simulink model "PR_controlv8planning"  (R2024a)
settings: Solver=VariableStepAuto  StartTime=0.0  StopTime=stoptime  RelTol=1e-3
values from neighbouring files (symbols this model uses):
  amp_factor = 0.01    [find_different_length_masses.m]    (also in find_different_length_masses_noretrain.m; find_good_reservoirs.m; plot_angle.m)
  rc = ESN_trainbysim(Nr, 'sizeinput', sizeinput, 'nodenuminput', 3, 'sizeoutput', sizeoutput,              'timeConst', timeConstant, 'spectralRadius', SR, 'inputScaling', 1, 'connectivity', 0.5, 'biasScaling', 0,              'regularization', 1e-1, 'delaylen', 0.1, 'timestep', 0.01, 'normmethod', normmethod, 'ifxnorm', ifxnorm, 'sizereadout', Nr + sizeinput + 1)    [find_different_length_masses.m]    (also in find_different_length_masses_noretrain.m; find_good_reservoirs.m = ESN_trainbysim(Nr, 'sizeinput', sizeinput, 'nodenuminput', 3; plot_angle.m)
  robot_pendepth = 0.02    [find_different_length_masses.m]    (also in find_different_length_masses_noretrain.m; find_good_reservoirs.m; plot_angle.m)
  robot_penlength = 0.2    [find_different_length_masses.m]    (also in find_different_length_masses_noretrain.m; find_good_reservoirs.m; plot_angle.m = 0.1)
  robot_penwidth = 0.02    [find_different_length_masses.m]    (also in find_different_length_masses_noretrain.m; find_good_reservoirs.m; plot_angle.m)
  robot_sphere_mass = 0.1    [find_different_length_masses.m]    (also in find_different_length_masses_noretrain.m; find_good_reservoirs.m; plot_angle.m)
  samplingrate = 0.01    [find_different_length_masses.m]    (also in find_different_length_masses_noretrain.m; find_good_reservoirs.m; plot_angle.m; stmpcevaluation.m)
  torquelim = fraction*mass*robot_penlength    (= 0.05)    [find_different_length_masses.m]    (also in find_different_length_masses_noretrain.m; find_good_reservoirs.m; plot_angle.m)
  Win = eye(2)    [find_different_length_masses.m]    (also in find_different_length_masses_noretrain.m; find_good_reservoirs.m; plot_angle.m; stmpcevaluation.m)
  X = esn.train_reservoirReadoutWashed    [ESN_trainbysim.m]
  Y = esn.train_reservoirTargetWashed{i}    [ESN_trainbysim.m]
undefined symbols (not defined in the file or in its folder): arm_radius, arm_radius_previus, spring_position_scale, Z
libraries: sm_lib x9, nesl_utility x5, dspindex x1
settings Model: Creator=fy264  LastModifiedBy=fy264
settings OptimizationCC: ReuseModelBlockBuffer=off
settings DebuggingCC: AlgebraicLoopMsg=none  ArtificialAlgebraicLoopMsg=none
settings RTWCC: GPUComputeCapability=3.5

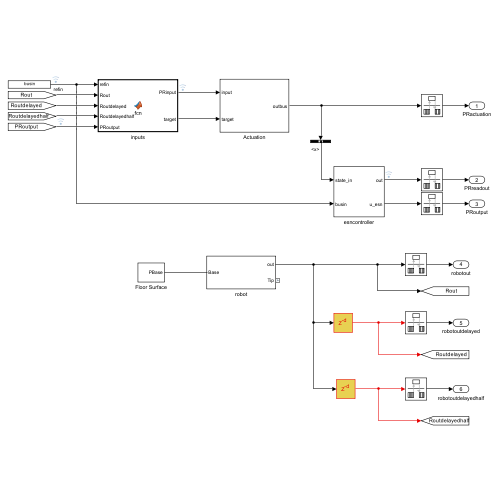
[thumbnail: Simulink's stored preview of the top-level diagram]
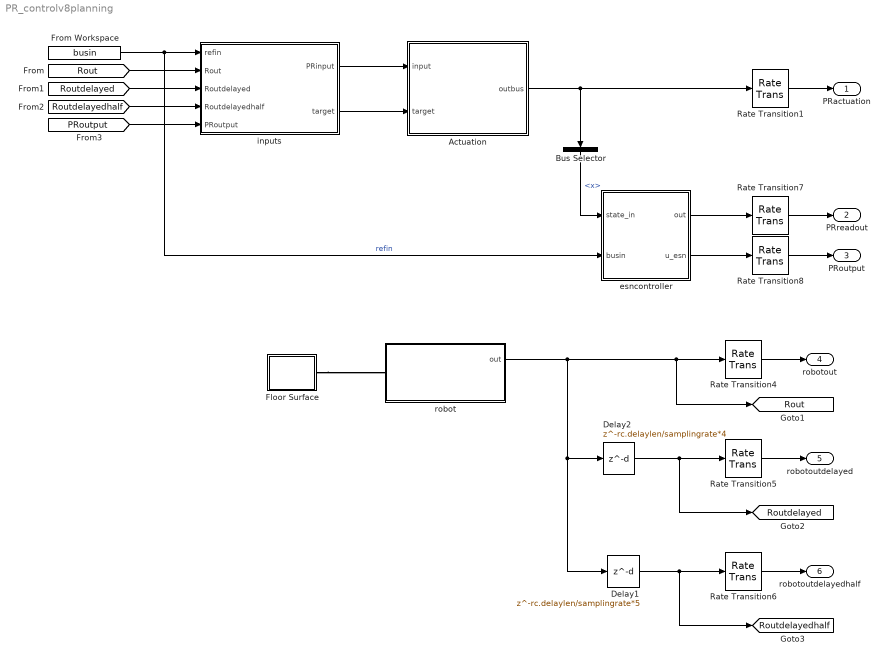
== system PR_controlv8planning ==
  Actuation : Subsystem  mask{xnorm=rc.xnorm}
  Bus Selector : BusSelector  OutputSignals=x
  Delay1 : Delay  DelayLength=rc.delaylen/samplingrate*5  InitialCondition=0
  Delay2 : Delay  DelayLength=rc.delaylen/samplingrate*4  InitialCondition=0
  Floor Surface : Subsystem  mask{length=0.5, width=0.5}
      mask prompts: length "grid length [m]"; width "grid width [m]"
  From Workspace : FromWorkspace  VariableName=busin  OutDataTypeStr=Bus: SinusoidBus  OutputAfterFinalValue=Holding final value
  Rate Transition{1,4..8} (6 alike) : RateTransition  OutPortSampleTime=samplingrate
  esncontroller : Subsystem  mask{Nr=rc.Nr, tau=rc.tau, Win=rc.Win, Wb=rc.Wb, Wr=rc.Wr, sizeinput=rc.sizeinput, nodenuminput=rc.nodenuminput, timestep=rc.timestep, ini_S=rc.initialstate, delaylen=rc.delaylen, delaynorm=rc.delaynorm, normmethod=rc.normmethod, ifxnorm=rc.ifxnorm, xnorm=rc.xnorm, Wout=0}
      mask prompts: delaynorm "delaynrom"
  inputs : MATLAB Function  TreatAsAtomicUnit=on
  robot : Subsystem
  PRactuation : Outport
  PRreadout : Outport  Port=2
  PRoutput : Outport  Port=3
  robotout : Outport  Port=4
  robotoutdelayed : Outport  Port=5
  robotoutdelayedhalf : Outport  Port=6
  tag scope: Rout=global, Routdelayed=global, Routdelayedhalf=global
  wires:
  Actuation/1(outbus) -> Bus Selector/1, Rate Transition1/1
  Rate Transition1/1 -> PRactuation/1
  Rate Transition4/1 -> robotout/1
  inputs/1(PRinput) -> Actuation/1(input)
  From Workspace/1 -> esncontroller/2(busin), inputs/1(refin)  "refin"
  [Rout] -> inputs/2(Rout)
  Rate Transition5/1 -> robotoutdelayed/1
  robot/1(out) -> Delay2/1, Delay1/1, Rate Transition4/1, [Rout]
  Delay2/1 -> [Routdelayed], Rate Transition5/1
  [Routdelayed] -> inputs/3(Routdelayed)
  inputs/2(target) -> Actuation/2(target)
  Delay1/1 -> [Routdelayedhalf], Rate Transition6/1
  Rate Transition6/1 -> robotoutdelayedhalf/1
  [Routdelayedhalf] -> inputs/4(Routdelayedhalf)
  esncontroller/2(u_esn) -> Rate Transition8/1
  Bus Selector/1 -> esncontroller/1(state_in)  "<x>"
  esncontroller/1(out) -> Rate Transition7/1
  Rate Transition7/1 -> PRreadout/1
  Rate Transition8/1 -> PRoutput/1
  [PRoutput] -> inputs/5(PRoutput)
  connections:
  Floor Surface/RConn1 -- robot/LConn1

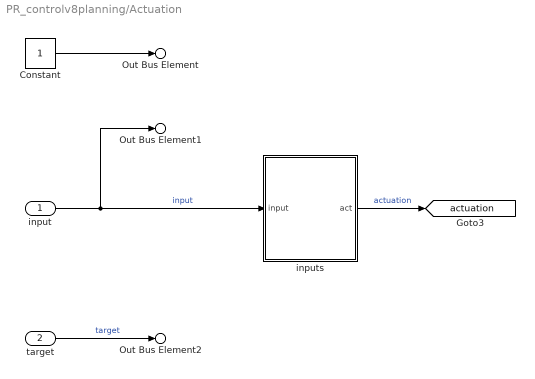
== system PR_controlv8planning/Actuation ==
  input : Inport
  target : Inport  Port=2
  Constant : Constant
  inputs : MATLAB Function  TreatAsAtomicUnit=on
  Out Bus Element : Outport  PortName=outbus  Element=const
  Out Bus Element1 : Outport  PortName=outbus  Element=x
  Out Bus Element2 : Outport  PortName=outbus  Element=target
  tag scope: actuation=global
  wires:
  input/1 -> Out Bus Element1/1, inputs/1(input)  "input"
  inputs/1(act) -> [actuation]  "actuation"
  Constant/1 -> Out Bus Element/1
  target/1 -> Out Bus Element2/1  "target"

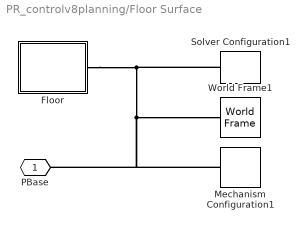
== system PR_controlv8planning/Floor Surface ==
  Floor : Subsystem
  Mechanism Configuration1 : sm_lib/Utilities/Mechanism Configuration  UniformGravity=Constant  GravityVector=[0 0 -9.80665]  GravityVectorUnits=m/s^2  LinearizationDelta=0.001  JointModeTransitionNonlinearIterations=2
  Solver Configuration1 : nesl_utility/Solver Configuration  PhysicalDomain=network_engine_domain  SubClassName=solver  LeftPortType=input  RightPortType=generic  Tones=[]  Harmonics=[]  SimulateNoise=off  Profile=off  UseLocalSampling=off  EnableSwitchedLinearOptims=on  FrequencyDomain=off  UseCCode=off  RelTol=0.001  AbsTol=1e-06  MinStep=1e-09  ToWorkspace=off  RevertToSquareIcSolve=off  NumHomotopyIterations=100  PhasorMode=off  PhasorModeNumHarmonics=1  ConsistencySolver=NEWTON_FTOL  IndexReductionMethod=DerivativeReplacement  DoDC=off  ResidualTolerance=1e-09  ConsistencyTolSource=GLOBAL  ConsistencyAbsTol=0.001  ConsistencyRelTol=0.001  ConsistencyTolFactor=0.001  UseLocalSolver=off  LocalSolverChoice=NE_BACKWARD_EULER_ADVANCER  ResolveIndetEquations=on  FunctionEvalNumThread=1  LocalSolverSampleTime=0.0002  DoFixedCost=off  MaxNonlinIter=10  MaxModeIter=2  ComputeImpulses=off  ImpulseIterations=2  LinearAlgebra=Sparse  LinearAlgebraNumThread=0  EquationFormulation=NE_TIME_EF  DelaysMemoryBudget=1024  AutomaticFiltering=off  FilteringTimeConstant=0.001  PartitionStorageMethod=AS_NEEDED  PartitionMemoryBudget=1024  PartitionMethod=FAST  MultibodyUseLocalSolver=off  MultibodyLocalSolverChoice=ODE1  MultibodyLocalSolverSampleTime=0.001
  World Frame1 : sm_lib/Frames and Transforms/World Frame
  PBase : PMIOPort  Side=Right
  connections:
  Floor/RConn1 -- PBase/RConn1 -- Mechanism Configuration1/RConn1 -- World Frame1/RConn1 -- Solver Configuration1/RConn1

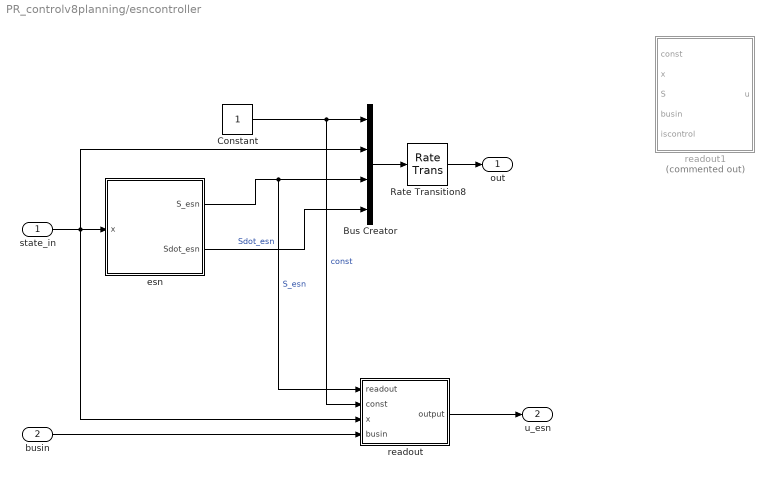
== system PR_controlv8planning/esncontroller ==
  state_in : Inport
  busin : Inport  Port=2
  Bus Creator : BusCreator  Inputs=4
  Constant : Constant
  Rate Transition8 : RateTransition  OutPortSampleTime=timestep
  esn : Subsystem  mask{Nr=rc.Nr, sizeinput=rc.sizeinput, nodenuminput=rc.nodenuminput, Win=rc.Win, Wr=rc.Wr, Wb=rc.Wb, tau=rc.tau, timestep=rc.timestep, ini_S=rc.initialstate}
  readout : Subsystem  mask{Woutmat=rc.Woutmat}
  readout1 : MATLAB Function  Commented=on  TreatAsAtomicUnit=on
  out : Outport
  u_esn : Outport  Port=2
  wires:
  Bus Creator/1 -> Rate Transition8/1
  Rate Transition8/1 -> out/1
  esn/2(Sdot_esn) -> Bus Creator/4  "Sdot_esn"
  esn/1(S_esn) -> readout/1(readout), Bus Creator/3  "S_esn"
  Constant/1 -> readout/2(const), Bus Creator/1  "const"
  state_in/1 -> readout/3(x), esn/1(x), Bus Creator/2
  busin/1 -> readout/4(busin)
  readout/1(output) -> u_esn/1

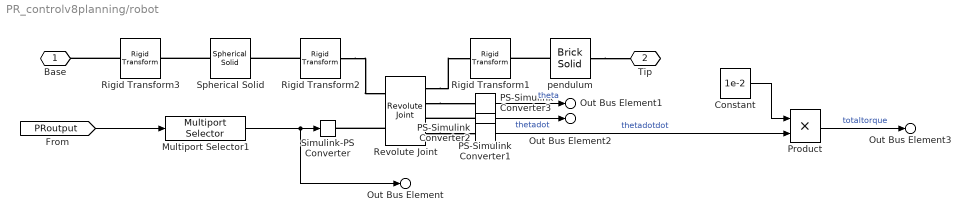
== system PR_controlv8planning/robot ==
  Constant : Constant  Value=1e-2
  Multiport Selector1 : dspindex/Multiport Selector  rowsOrCols=Rows  idxCellArray=1  idxErrMode=Clip Index
  PS-Simulink Converter1 : nesl_utility/PS-Simulink Converter  PhysicalDomain=network_engine_domain  SubClassName=ps_output  LeftPortType=input  RightPortType=output  PseudoPeriodic=off  Frequencies=[]  VectorFormat=1-D array  Unit=1  AffineConversion=off
  PS-Simulink Converter2 : nesl_utility/PS-Simulink Converter  PhysicalDomain=network_engine_domain  SubClassName=ps_output  LeftPortType=input  RightPortType=output  PseudoPeriodic=off  Frequencies=[]  VectorFormat=1-D array  Unit=1  AffineConversion=off
  PS-Simulink Converter3 : nesl_utility/PS-Simulink Converter  PhysicalDomain=network_engine_domain  SubClassName=ps_output  LeftPortType=input  RightPortType=output  PseudoPeriodic=off  Frequencies=[]  VectorFormat=1-D array  Unit=1  AffineConversion=off
  Product : Product
  Revolute Joint : sm_lib/Joints/Revolute Joint  JointMode=Normal  CompositeWrenchDir=FollowerOnBase  CompositeWrenchFrame=BaseFrame  SenseConstraintForce=off  SenseConstraintTorque=off  SenseTotalForce=off  SenseTotalTorque=off  PositionTargetSpecify=on  PositionTargetPriority=Low  PositionTargetValue=robot_ini_theta_p  PositionTargetValueUnits=rad  VelocityTargetSpecify=on  VelocityTargetPriority=Low  VelocityTargetValue=robot_ini_thetadot_p  VelocityTargetValueUnits=rad/s  EquilibriumPosition=0  EquilibriumPositionUnits=rad  SpringStiffness=0  SpringStiffnessUnits=N*m/rad  DampingCoefficient=robot_damping_coeff  DampingCoefficientUnits=N*m/(rad/s)  LowerLimitSpecify=off  LowerLimitBound=-90  LowerLimitBoundUnits=deg  LowerLimitStiffness=1e4  LowerLimitStiffnessUnits=N*m/deg  LowerLimitDamping=10  LowerLimitDampingUnits=N*m/(deg/s)  LowerLimitTransitionRegionWidth=0.1  LowerLimitTransitionRegionWidthUnits=deg  UpperLimitSpecify=off  UpperLimitBound=90  UpperLimitBoundUnits=deg  UpperLimitStiffness=1e4  UpperLimitStiffnessUnits=N*m/deg  UpperLimitDamping=10  UpperLimitDampingUnits=N*m/(deg/s)  UpperLimitTransitionRegionWidth=0.1  UpperLimitTransitionRegionWidthUnits=deg  TorqueActuationMode=InputTorque  MotionActuationMode=ComputedMotion  SensePosition=on  SenseVelocity=on  SenseAcceleration=on  SenseTorqueForce=off  SenseLowerLimitTorqueForce=off  SenseUpperLimitTorqueForce=off
  Rigid Transform1 : sm_lib/Frames and Transforms/Rigid Transform  RotationMethod=AlignedAxes  FollAlignAxisA=+X  BaseAlignAxisA=+X  FollAlignAxisB=-Z  BaseAlignAxisB=+Y  RotationStandardAxis=+Z  RotationAngle=180  RotationAngleUnits=deg  RotationArbitraryAxis=[0 0 1]  RotationSequenceAxes=FollowerAxes  RotationSequence=XYX  RotationSequenceAngles=[0 0 0]  RotationSequenceAnglesUnits=deg  RotationMatrix=[1 0 0; 0 1 0; 0 0 1]  Quaternion=[1 0 0 0]  TranslationMethod=None  TranslationCartesianOffset=[arm_radius*spring_position_scale 0 0]  TranslationCartesianOffsetUnits=m  TranslationStandardAxis=+Z  TranslationStandardOffset=0  TranslationStandardOffsetUnits=m  TranslationROffset=arm_radius_previus*spring_position_scale  TranslationROffsetUnits=m  TranslationThetaOffset=theta  TranslationThetaOffsetUnits=deg  TranslationZOffset=0  TranslationZOffsetUnits=m
  Rigid Transform2 : sm_lib/Frames and Transforms/Rigid Transform  RotationMethod=AlignedAxes  FollAlignAxisA=+X  BaseAlignAxisA=+X  FollAlignAxisB=+Y  BaseAlignAxisB=+Z  RotationStandardAxis=+Z  RotationAngle=180  RotationAngleUnits=deg  RotationArbitraryAxis=[0 0 1]  RotationSequenceAxes=FollowerAxes  RotationSequence=XYX  RotationSequenceAngles=[0 0 0]  RotationSequenceAnglesUnits=deg  RotationMatrix=[1 0 0; 0 1 0; 0 0 1]  Quaternion=[1 0 0 0]  TranslationMethod=None  TranslationCartesianOffset=[arm_radius*spring_position_scale 0 0]  TranslationCartesianOffsetUnits=m  TranslationStandardAxis=+Z  TranslationStandardOffset=0  TranslationStandardOffsetUnits=m  TranslationROffset=arm_radius_previus*spring_position_scale  TranslationROffsetUnits=m  TranslationThetaOffset=theta  TranslationThetaOffsetUnits=deg  TranslationZOffset=0  TranslationZOffsetUnits=m
  Rigid Transform3 : sm_lib/Frames and Transforms/Rigid Transform  RotationMethod=None  FollAlignAxisA=+X  BaseAlignAxisA=+X  FollAlignAxisB=+Y  BaseAlignAxisB=+Z  RotationStandardAxis=+Z  RotationAngle=180  RotationAngleUnits=deg  RotationArbitraryAxis=[0 0 1]  RotationSequenceAxes=FollowerAxes  RotationSequence=XYX  RotationSequenceAngles=[0 0 0]  RotationSequenceAnglesUnits=deg  RotationMatrix=[1 0 0; 0 1 0; 0 0 1]  Quaternion=[1 0 0 0]  TranslationMethod=StandardAxis  TranslationCartesianOffset=[arm_radius*spring_position_scale 0 0]  TranslationCartesianOffsetUnits=m  TranslationStandardAxis=+Z  TranslationStandardOffset=robot_penposz  TranslationStandardOffsetUnits=m  TranslationROffset=arm_radius_previus*spring_position_scale  TranslationROffsetUnits=m  TranslationThetaOffset=theta  TranslationThetaOffsetUnits=deg  TranslationZOffset=0  TranslationZOffsetUnits=m
  Simulink-PS Converter : nesl_utility/Simulink-PS Converter  PhysicalDomain=network_engine_domain  SubClassName=ps_input  LeftPortType=input  RightPortType=output  PseudoPeriodic=off  Frequencies=[]  NoiseDistribution=none  NoiseParameters=[]  Unit=1  AffineConversion=off  FilteringAndDerivatives=provide  SimscapeFilterOrder=1  InputFilterTimeConstant=0.001  UdotUserProvided=0
  Spherical Solid : sm_lib/Body Elements/Spherical Solid  SphereRadius=robot_sphere_radius  SphereRadiusUnits=m  ExportEntireGeometry=off  InertiaType=CalculateFromGeometry  BasedOnType=Mass  Density=1000  DensityUnits=kg/m^3  Mass=robot_sphere_mass  MassUnits=kg  CenterOfMass=[0 0 0]  CenterOfMassUnits=m  MomentsOfInertia=[1 1 1]  MomentsOfInertiaUnits=kg*m^2  ProductsOfInertia=[0 0 0]  ProductsOfInertiaUnits=kg*m^2  GraphicType=FromGeometry  MarkerShape=Sphere  MarkerSize=10  GraphicVisPropType=SimpleVisualProperties  GraphicDiffuseColor=[1.0 0.0 0.0]  GraphicOpacity=1.0  GraphicSpecularColor=[0.5 0.5 0.5 1.0]  GraphicAmbientColor=[0.15 0.15 0.15 1.0]  GraphicEmissiveColor=[0.0 0.0 0.0 1.0]  GraphicShininess=75  DoExposeReferenceFrame=on  SerializedFrames=<Frames><Frame><Id>Frame1</Id><Value><Name>F1</Name><Origin><Source>ReferenceFrame</Source><FeatureName></FeatureName></Origin><PrimaryAxis><DefinedDirection>+Z</DefinedDirection><Source>ReferenceFrame</Source><SourceDirection>+Z</SourceDirection><FeatureName></FeatureName></PrimaryAxis><SecondaryAxis><DefinedDirection>+X</DefinedDirection><Source>ReferenceFrame</Source><SourceDirection>+X</SourceDirection><FeatureName></FeatureName></SecondaryAxis></Value></Frame></Frames>
  pendulum : sm_lib/Body Elements/Brick Solid  BrickDimensions=[robot_penwidth robot_pendepth robot_penlength]  BrickDimensionsUnits=m  ExportEntireGeometry=off  InertiaType=CalculateFromGeometry  BasedOnType=Density  Density=robot_penrho  DensityUnits=kg/m^3  Mass=1  MassUnits=kg  CenterOfMass=[0 0 0]  CenterOfMassUnits=m  MomentsOfInertia=[1 1 1]  MomentsOfInertiaUnits=kg*m^2  ProductsOfInertia=[0 0 0]  ProductsOfInertiaUnits=kg*m^2  GraphicType=FromGeometry  MarkerShape=Sphere  MarkerSize=10  GraphicVisPropType=SimpleVisualProperties  GraphicDiffuseColor=[1.0 0.0 1.0]  GraphicOpacity=1.0  GraphicSpecularColor=[0.5 0.5 0.5 1.0]  GraphicAmbientColor=[0.15 0.15 0.15 1.0]  GraphicEmissiveColor=[0.0 0.0 0.0 1.0]  GraphicShininess=75  DoExposeReferenceFrame=off  SerializedFrames=<Frames><Frame><Id>Frame1</Id><Value><Name>F1</Name><Origin><Source>GeometricFeature</Source><FeatureName>-z surface</FeatureName></Origin><PrimaryAxis><DefinedDirection>+Z</DefinedDirection><Source>ReferenceFrame</Source><SourceDirection>+Z</SourceDirection><FeatureName></FeatureName></PrimaryAxis><SecondaryAxis><DefinedDirection>+X</DefinedDirection><Source>ReferenceFrame</Source><SourceDirection>+X</SourceDirection><FeatureName></FeatureName></SecondaryAxis></Value></Frame><Frame><Id>Frame2</Id><Value><Name>F2</Name><Origin><Source>GeometricFeature</Source><FeatureName>+z surface</FeatureName></Origin><PrimaryAxis><DefinedDirection>+Z</DefinedDirection><Source>ReferenceFrame</Source><SourceDirection>-Z</SourceDirection><FeatureName></FeatureName></PrimaryAxis><SecondaryAxis><DefinedDirection>+X</DefinedDirection><Source>ReferenceFrame</Source><SourceDirection>+X</SourceDirection><FeatureName></FeatureName></SecondaryAxis></Value></Frame></Frames>
  Base : PMIOPort  Side=Left
  Tip : PMIOPort  Port=2  Side=Right
  Out Bus Element1 : Outport  PortName=out  Element=theta
  Out Bus Element2 : Outport  PortName=out  Element=thetadot
  Out Bus Element3 : Outport  PortName=out  Element=totaltorque
  Out Bus Element : Outport  PortName=out  Element=actuationtorque
  wires:
  PS-Simulink Converter3/1 -> Out Bus Element1/1  "theta"
  PS-Simulink Converter1/1 -> Out Bus Element2/1  "thetadot"
  PS-Simulink Converter2/1 -> Product/2  "thetadotdot"
  Product/1 -> Out Bus Element3/1  "totaltorque"
  Constant/1 -> Product/1
  Multiport Selector1/1 -> Simulink-PS Converter/1, Out Bus Element/1
  [PRoutput] -> Multiport Selector1/1
  connections:
  Revolute Joint/LConn2 -- Simulink-PS Converter/RConn1
  Revolute Joint/RConn2 -- PS-Simulink Converter3/LConn1
  Rigid Transform2/LConn1 -- Spherical Solid/RConn1
  PS-Simulink Converter1/LConn1 -- Revolute Joint/RConn3
  Spherical Solid/LConn1 -- Rigid Transform3/RConn1
  pendulum/LConn1 -- Rigid Transform1/RConn1
  Rigid Transform3/LConn1 -- Base/RConn1
  pendulum/RConn1 -- Tip/RConn1
  Rigid Transform2/RConn1 -- Revolute Joint/LConn1
  Revolute Joint/RConn4 -- PS-Simulink Converter2/LConn1
  Revolute Joint/RConn1 -- Rigid Transform1/LConn1

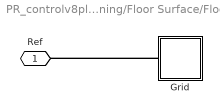
== system PR_controlv8planning/Floor Surface/Floor ==
  Grid : Subsystem  mask(Grid Lines){grid_origin=[-length -width 0], grid_size=[length width], grid_linewidth=0.001, grid_num_squares=20, grid_color=[0.8 0.8 0.8], grid_opacity=0.8}
      mask prompts: grid_origin "Origin (m)"; grid_size "Arena size (m)"; grid_linewidth "Grid Line Width (m)"; grid_num_squares "Number of Squares"; grid_color "Grid Color [RGB]"; grid_opacity "Grid Opacity (0-1)"
      mask help: Creates grids on 3 planes XZ, YZ, and XZ.
      mask init:
      | mesh_xsec = Extr_Data_Mesh(grid_size(1), grid_size(2), grid_num_squares, grid_num_squares, grid_size(1)/grid_num_squares-grid_linewidth, grid_size(2)/grid_num_squares-grid_linewidth);
  Ref : PMIOPort  Side=Right
  connections:
  Grid/LConn1 -- Ref/RConn1

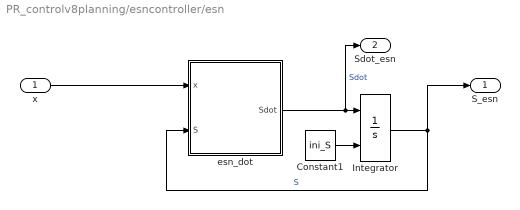
== system PR_controlv8planning/esncontroller/esn ==
  x : Inport
  Constant1 : Constant  Value=ini_S  VectorParams1D=off
  Integrator : Integrator  InitialConditionSource=external
  esn_dot : MATLAB Function  TreatAsAtomicUnit=on
  S_esn : Outport
  Sdot_esn : Outport  Port=2
  wires:
  esn_dot/1(Sdot) -> Sdot_esn/1, Integrator/1  "Sdot"
  Integrator/1 -> S_esn/1, esn_dot/2(S)  "S"
  Constant1/1 -> Integrator/2
  x/1 -> esn_dot/1(x)

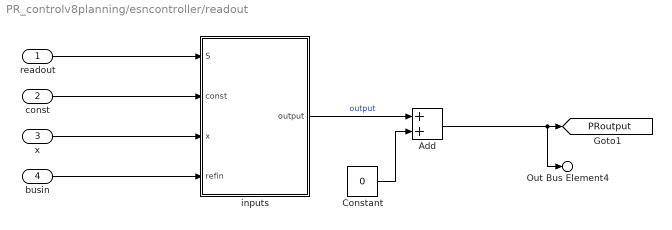
== system PR_controlv8planning/esncontroller/readout ==
  readout : Inport
  const : Inport  Port=2
  x : Inport  Port=3
  busin : Inport  Port=4
  Add : Sum
  Constant : Constant  Value=0
  inputs : MATLAB Function  TreatAsAtomicUnit=on
  Out Bus Element4 : Outport  PortName=output  Element=output
  tag scope: PRoutput=global
  wires:
  readout/1 -> inputs/1(S)
  const/1 -> inputs/2(const)
  x/1 -> inputs/3(x)
  inputs/1(output) -> Add/1  "output"
  Constant/1 -> Add/2
  Add/1 -> Out Bus Element4/1, [PRoutput]
  busin/1 -> inputs/4(refin)

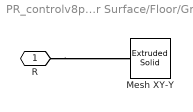
== system PR_controlv8planning/Floor Surface/Floor/Grid ==
  Mesh XY-Y : sm_lib/Body Elements/Extruded Solid  ExtrusionType=General  PolygonNumSides=3  PolygonOuterRadius=1  PolygonOuterRadiusUnits=m  ExportEntireGeometry=off  ExtrusionCrossSection=mesh_xsec  ExtrusionCrossSectionUnits=m  ExportConvexHullGeometry=off  ExtrusionLength=grid_linewidth  ExtrusionLengthUnits=m  InertiaType=CalculateFromGeometry  BasedOnType=Density  Density=1000  DensityUnits=kg/(m^3)  Mass=1  MassUnits=kg  CenterOfMass=[0 0 0]  CenterOfMassUnits=m  MomentsOfInertia=[1 1 1]  MomentsOfInertiaUnits=kg*m^2  ProductsOfInertia=[0 0 0]  ProductsOfInertiaUnits=kg*m^2  GraphicType=FromGeometry  MarkerShape=Sphere  MarkerSize=10  GraphicVisPropType=SimpleVisualProperties  GraphicDiffuseColor=[0.5 0.5 0.5]  GraphicOpacity=1.0  GraphicSpecularColor=[0.5 0.5 0.5 1.0]  GraphicAmbientColor=[0.15 0.15 0.15 1.0]  GraphicEmissiveColor=[0.0 0.0 0.0 1.0]  GraphicShininess=75  DoExposeReferenceFrame=on  SerializedFrames=<Frames/>
  R : PMIOPort  Side=Left
  connections:
  R/RConn1 -- Mesh XY-Y/RConn1

== matlab function PR_controlv8planning/Actuation/inputs ==
  data: input input; act output; Win parameter; xnorm parameter; amp_factor parameter
function act = fcn(input, Win, xnorm, amp_factor)

input = input(1:2)./xnorm(1:2);
inputmat = amp_factor.*[input 0.*input];

act = Win*inputmat;
end

== matlab function PR_controlv8planning/inputs ==
  data: refin input; PRinput output; Rout input; Routdelayed input; Routdelayedhalf input; PRoutput input; iscontrol parameter; target output
function [PRinput,target] = fcn(refin, Rout, Routdelayed, Routdelayedhalf, PRoutput, iscontrol)

if iscontrol
    PRinput = [Rout(1);
        Rout(2);
        PRoutput(2);
        PRoutput(3);
        refin.x1;
        refin.x2];
else
    PRinput = [Routdelayedhalf(1);
        Routdelayedhalf(2);
        Routdelayed(1);
        Routdelayed(2);
        Rout(1);
        Rout(2)];
end
target = [Routdelayedhalf(3);
    Routdelayed(1);
    Routdelayed(2)];

end

== matlab function PR_controlv8planning/esncontroller/esn/esn_dot ==
  data: x input; Sdot output; S input; Nr parameter; sizeinput parameter; nodenuminput parameter; Win parameter; Wr parameter; Wb parameter; tau parameter
function Sdot = fcn(x, S, Nr, sizeinput, nodenuminput, Win, Wr, Wb, tau)

x = x(1:2);
u = zeros(Nr, 1);
% 
% for i = 1:Nr
%     u(i) = x(mod(i-1, 2) + 1);
% end
% %u = [x(1); 0; x(2); 0];

u(1:Nr/2) = x(1);
u(Nr/2+1:Nr) = x(2);

Sdot = (-S + tanh(Win.*u + Wr*S + Wb))/tau;

end

== matlab function PR_controlv8planning/esncontroller/readout1 ==
  data: const input; u output; x input; S input; busin input; Wout parameter; iscontrol input
function u = fcn(const, x, S, busin, Wout,  iscontrol)
if iscontrol
    disp("Here")
    readout = [const;x;S];
    u = Wout*readout;
else
    disp('Here')
    u = 0;


end

== matlab function PR_controlv8planning/esncontroller/readout/inputs ==
  data: S input; const input; x input; refin input; output output size=3; Woutmat parameter; torquelim parameter
function output = fcn(S, const, x, refin, Woutmat, torquelim)

readoutt = [const; x; S];
output = Woutmat*readoutt;

if output(1) > torquelim
    output(1) = torquelim;
elseif output(1) < -torquelim
    output(1) = -torquelim;
end

if abs(output(2) - refin.x1) < pi/4
    output(2) = refin.x1;
    output(3) = refin.x2;
end

end
